simulink model "iplimage_io"  (Simulink 10.1)
settings: Solver=FixedStepDiscrete  StartTime=0.0  StopTime=10.0  RelTol=1e-3  EnableMultiTasking=on
settings Model: Creator=Demo  LastModifiedBy=MaximeBe
settings DataIOCC: LimitDataPoints=on  SaveFormat=Dataset
settings OptimizationCC: ZeroExternalMemoryAtStartup=off  ZeroInternalMemoryAtStartup=off  LifeSpan=auto
settings DebuggingCC: UnderspecifiedInitializationDetection=Simplified  MergeDetectMultiDrivingBlocksExec=error  AllowSymbolicDim=off  SFExecutionAtInitializationDiag=warning
settings HardwareCC: ProdBitPerPointer=64  ProdBitPerSizeT=64  ProdBitPerPtrDiffT=64  ProdLargestAtomicFloat=Float  ProdIntDivRoundTo=Zero  ProdEndianess=LittleEndian  ProdWordSize=64  ProdHWDeviceType=Intel->x86-64 (Windows64)
settings RTWCC: Description=Generate an RTMaps component embedding the model  SystemTargetFile=rtmaps.tlc  TemplateMakefile=rtmaps_default_tmf  PostCodeGenCommand=rtmaps_post_code_generation(buildInfo)  RetainRTWFile=on  TargetLang=C++
settings STFCustomTargetCC: ModelReferenceCompliant=off  ConcurrentExecutionCompliant=on  CombineOutputUpdateFcns=on  MultiInstanceERTCode=on  CodeInterfacePackaging=C++ class  CPPClassGenCompliant=on  GRTInterface=off  SystemTargetFile=rtmaps.tlc
settings GRTTargetCC: ModelReferenceCompliant=off  ParMdlRefBuildCompliant=off  CompOptLevelCompliant=off  CombineOutputUpdateFcns=on  MatFileLogging=off  MultiInstanceERTCode=on  CodeInterfacePackaging=C++ class  GRTInterface=off  UseToolchainInfoCompliant=off
settings CPPComponent: GenerateDestructor=on  ExternalIOMemberVisibility=private  GenerateExternalIOAccessMethods=Inlined structure-based method  ParameterMemberVisibility=public  InternalMemberVisibility=private  GenerateParameterAccessMethods=None  GenerateInternalMemberAccessMethods=None  UseOperatorNewForModelRefRegistration=off  IncludeModelTypesInModelClass=on

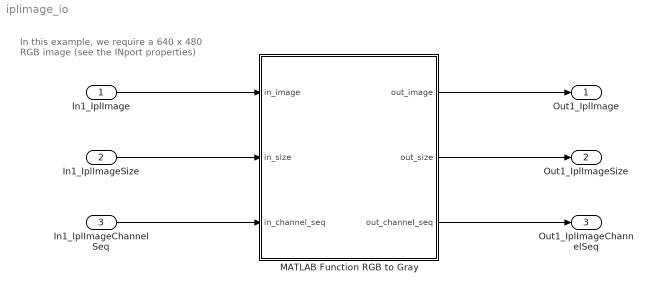
== system iplimage_io ==
  note: In this example, we require a
      | 640 x 480 RGB image
      | (see the INport properties)
  In1_IplImage : Inport  OutDataTypeStr=uint8  PortDimensions=[640 480 3]
  In1_IplImageSize : Inport  Port=2  OutDataTypeStr=int32  PortDimensions=2
  In1_IplImageChannelSeq : Inport  Port=3  PortDimensions=4
  MATLAB Function RGB to Gray : MATLAB Function  TreatAsAtomicUnit=on
  Out1_IplImage : Outport
  Out1_IplImageSize : Outport  Port=2
  Out1_IplImageChannelSeq : Outport  Port=3
  wires:
  In1_IplImage/1 -> MATLAB Function RGB to Gray/1(in_image)
  In1_IplImageSize/1 -> MATLAB Function RGB to Gray/2(in_size)
  MATLAB Function RGB to Gray/1(out_image) -> Out1_IplImage/1
  MATLAB Function RGB to Gray/3(out_channel_seq) -> Out1_IplImageChannelSeq/1
  MATLAB Function RGB to Gray/2(out_size) -> Out1_IplImageSize/1
  In1_IplImageChannelSeq/1 -> MATLAB Function RGB to Gray/3(in_channel_seq)

== matlab function MATLAB Function RGB to Gray ==
  data: in_image input double; out_image output uint8; out_size output double; in_size input double; in_channel_seq input double; out_channel_seq output double
function [out_image, out_size, out_channel_seq] = fcn(in_image, in_size, in_channel_seq)
%#codegen

height =  in_size(1);
width  =  in_size(2);

out_image = rgb2gray(in_image);
%out_image = edge(rgb2gray(in_image), 'Canny');  % requires the image processing toolbox

out_size        = int32([height width]);  % must be a 2-element int32 array
out_channel_seq = uint8('GRAY');  % must be a 4-element uint8 array
